simulink model "backwardfault"  (Simulink 8.5)
settings: Solver=ode23tb  SolverMode=SingleTasking  StartTime=0.0  StopTime=0.15  RelTol=1e-3  AbsTol=20e-6
libraries: powerlib x28
settings Model: Creator=Dr. Lotfifard  LastModifiedBy=PC  ExtModeTrigMode=oneshot  ExtModeArmWhenConnect=off
settings SolverCC: MaxOrder=2
settings OptimizationCC: BlockReduction=off  BooleanDataType=off
settings DebuggingCC: SaveWithParameterizedLinksMsg=none  SignalResolutionControl=TryResolveAllWithWarning  MultiTaskDSMMsg=warning  MultiTaskCondExecSysMsg=none  FcnCallInpInsideContextMsg=UseLocalSettings
settings HardwareCC: TargetUnknown=on
settings RTWCC: TemplateMakefile=grt_unix.tmf

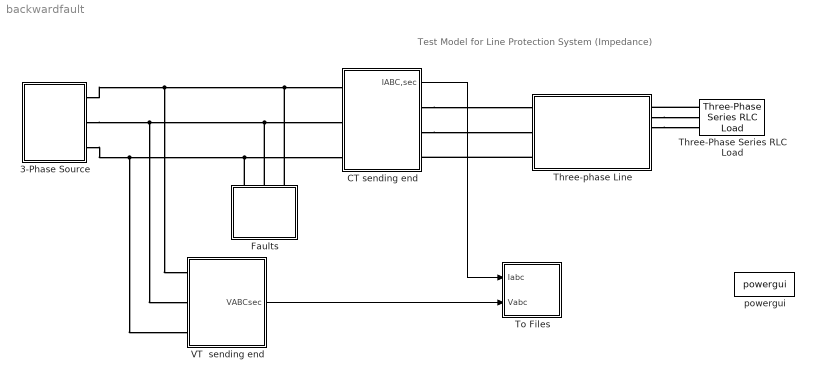
== system backwardfault ==
  note: Test Model for Line Protection System (Impedance)
  3-Phase Source : Subsystem  mask(Three-phase Source){Vrms=1000}
      mask prompts: Vrms "RMS Voltage for each phase"
      mask Display: plot(0,0,100,100,[60,56,50,44,40,36,30,24,20],[50,40,33,40,50,60,66,60,50],[15,20,30,40,50,60,65,60,50,40,30,20,15],[50,35,27,25,26,35,50,65,73,76,73,65,50],[40,40],[90,76],[40,40],[10,25],[60,60],[75,87],[53,67],[79,79])
  CT sending end : Subsystem  mask{TC=1.2}
      mask prompts: TC "Maximum Normal Current"
  Faults : Subsystem  mask{tof='A-G', ft=0.05, RF=1e-6}
      mask prompts: tof "Type of fault"; ft "Fault time (in sec.)"; RF "Fault Resistance RF (in ohms)"
      mask init:
      | switch tof,
      |    case 1,
      |       %No faults or Normal
      |       S1=0;S2=0;S3=0;S4=0;
      |    case 2,
      |       %Fault A-G
      |       S1=1;S2=0;S3=0;S4=1;
      |    case 3,
      |       %Fault B-G
      |       S1=0;S2=1;S3=0;S4=1;
      |    case 4,
      |       %Fault B-G
      |       S1=0;S2=0;S3=1;S4=1;
      |    case 5,
      |       %Fault B-C
      |       S1=0;S2=1;S3=1;S4=0;
      |    case 6,
      |       %Fault A-C
      |       S1=1;S2=0;S3=1;S4=0;
      |    case 7,
      |       %Fault A-B
      |       S1=1;S2=1;S3=0;S4=0;
      |    case 8,
      |       %Fault A-B-C
      |       S1=1;S2=1;S3=1;S4=0;
      |    case 9,
      |       %Fault B-C-G
      |       S1=0;S2=1;S3=1;S4=1;
      |    case 10,
      |       %Fault A-C-G
      |       S1=1;S2=0;S3=1;S4=1;
      |    case 11,
      |       %Fault A-B-G
      |       S1=1;S2=1;S3=0;S4=1;
      |    case 12,
      |       %Fault A-B-C-G
      |       S1=1;S2=1;S3=1;S4=1;
      |    end;
      mask TypeOptions tof: 'Normal' | 'A-G' | 'B-G' | 'C-G' | 'B-C' | 'A-C' | 'A-B' | 'A-B-C' | 'B-C-G' | 'A-C-G' | 'A-B-G' | 'A-B-C-G'
      mask Display: plot(0,0,100,100,[44,47,56,38,50],[23,8,64,44,97],[56,47],[25,8])
  Three-Phase Series RLC Load : powerlib/Elements/Three-Phase Series RLC Load  LConnTagsString=A|B|C  Configuration=Y (grounded)  NominalVoltage=1000  NominalFrequency=60  ActivePower=10e3  InductivePower=100  CapacitivePower=100  Measurements=None  LoadType=constant Z
  Three-phase Line : Subsystem  mask(Three-pase Line){KM=50}
      mask prompts: KM "Fault location (1% to 99%) (the lenght of the line is 100 km):"
      mask Display: plot(0,0,100,100,[20,20,80,80,90,80,80,20,20,10],[50,40,40,50,50,50,61,61,50,50],[56,39],[55,55],[44,44],[44,55],[53,50,50],[44,48,55])
  To Files : Subsystem
  VT  sending end : Subsystem  mask{TP=1000}
      mask prompts: TP "Nominal Voltage,rms"
  powergui : powerlib/powergui  SimulationMode=Continuous  SolverType=Tustin/Backward Euler (TBE)  SampleTime=0  frequency=60  SPID=off  DisableSnubberDevices=off  DisableRonSwitches=off  DisableVfSwitches=off  SwTol=0  DisplayEquations=off  Interpol=off  methode=off  Ts=0  FunctionMessages=off  echomessages=off  HookPort=off  EnableUseOfTLC=off  x0status=blocks  frequencyindice=60  Pbase=100e6  ErrMax=1e-4  Iterations=50  UnitsV=kV  UnitsW=MW  buscounter=0  RestoreLinks=warning  ResistiveCurrentMeasurement=off  Frange=[0:2:500]  Ylog=off  Xlog=on  ShowGrid=off  save=off  variable=ZData  structure=0  ZoomFFT=on  StartTime=0.0  cycles=1  DisplayStyle=1  fundamental=60  FreqAxis=off  MaxFrequency=1000  frequencyindicesteady=1  RmsSteady=1  display=off
  wires:
  CT sending end/1(IABC,sec) -> To Files/1(Iabc)
  VT  sending end/1(VABCsec) -> To Files/2(Vabc)
  connections:
  3-Phase Source/RConn1 -- Faults/LConn3 -- CT sending end/LConn1 -- VT  sending end/LConn1
  3-Phase Source/RConn2 -- Faults/LConn2 -- CT sending end/LConn2 -- VT  sending end/LConn2
  3-Phase Source/RConn3 -- Faults/LConn1 -- CT sending end/LConn3 -- VT  sending end/LConn3
  Three-phase Line/LConn3 -- CT sending end/RConn3
  CT sending end/RConn2 -- Three-phase Line/LConn2
  CT sending end/RConn1 -- Three-phase Line/LConn1
  Three-Phase Series RLC Load/LConn1 -- Three-phase Line/RConn1
  Three-phase Line/RConn2 -- Three-Phase Series RLC Load/LConn2
  Three-phase Line/RConn3 -- Three-Phase Series RLC Load/LConn3

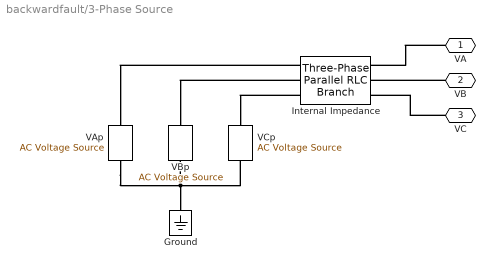
== system backwardfault/3-Phase Source ==
  Ground : powerlib/Elements/Ground  LConnTagsString=a
  Internal Impedance : powerlib/Elements/Three-Phase Parallel RLC Branch  LConnTagsString=A|B|C  RConnTagsString=A|B|C  BranchType=R  Resistance=1  Inductance=1e-3  Capacitance=1e-6  Measurements=None
  VAp : powerlib/Electrical Sources/AC Voltage Source  Amplitude=100  Phase=0  Frequency=60  SampleTime=0  Measurements=None
  VBp : powerlib/Electrical Sources/AC Voltage Source  Amplitude=100  Phase=0  Frequency=60  SampleTime=0  Measurements=None
  VCp : powerlib/Electrical Sources/AC Voltage Source  Amplitude=100  Phase=0  Frequency=60  SampleTime=0  Measurements=None
  VA : PMIOPort  Port=1  Side=Right
  VB : PMIOPort  Port=2  Side=Right
  VC : PMIOPort  Port=3  Side=Right
  connections:
  VAp/LConn1 -- VBp/LConn1 -- Ground/LConn1 -- VCp/LConn1
  Internal Impedance/LConn3 -- VCp/RConn1
  Internal Impedance/LConn2 -- VBp/RConn1
  Internal Impedance/LConn1 -- VAp/RConn1
  VA/RConn1 -- Internal Impedance/RConn1
  VB/RConn1 -- Internal Impedance/RConn2
  VC/RConn1 -- Internal Impedance/RConn3

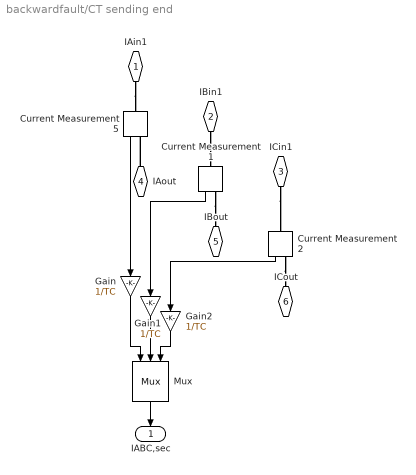
== system backwardfault/CT sending end ==
  Current Measurement1 : powerlib/Measurements/Current Measurement  PhasorSimulation=off  OutputType=Complex  PSBequivalent=0
  Current Measurement2 : powerlib/Measurements/Current Measurement  PhasorSimulation=off  OutputType=Complex  PSBequivalent=0
  Current Measurement5 : powerlib/Measurements/Current Measurement  PhasorSimulation=off  OutputType=Complex  PSBequivalent=0
  Gain : Gain  Gain=1/TC  SaturateOnIntegerOverflow=on  OutDataTypeStr=Inherit: Same as input  ParamDataTypeStr=Inherit: Same as input
  Gain1 : Gain  Gain=1/TC  SaturateOnIntegerOverflow=on  OutDataTypeStr=Inherit: Same as input  ParamDataTypeStr=Inherit: Same as input
  Gain2 : Gain  Gain=1/TC  SaturateOnIntegerOverflow=on  OutDataTypeStr=Inherit: Same as input  ParamDataTypeStr=Inherit: Same as input
  Mux : Mux  Inputs=3
  IAin1 : PMIOPort  Port=1  Side=Left
  IBin1 : PMIOPort  Port=2  Side=Left
  ICin1 : PMIOPort  Port=3  Side=Left
  IAout : PMIOPort  Port=4  Side=Right
  IBout : PMIOPort  Port=5  Side=Right
  ICout : PMIOPort  Port=6  Side=Right
  IABC,sec : Outport  InitialOutput=0
  wires:
  Mux/1 -> IABC,sec/1
  Current Measurement2/1 -> Gain2/1
  Gain/1 -> Mux/1
  Gain1/1 -> Mux/2
  Gain2/1 -> Mux/3
  Current Measurement1/1 -> Gain1/1
  Current Measurement5/1 -> Gain/1
  connections:
  IAin1/RConn1 -- Current Measurement5/LConn1
  ICin1/RConn1 -- Current Measurement2/LConn1
  IBin1/RConn1 -- Current Measurement1/LConn1
  IAout/RConn1 -- Current Measurement5/RConn1
  Current Measurement1/RConn1 -- IBout/RConn1
  Current Measurement2/RConn1 -- ICout/RConn1

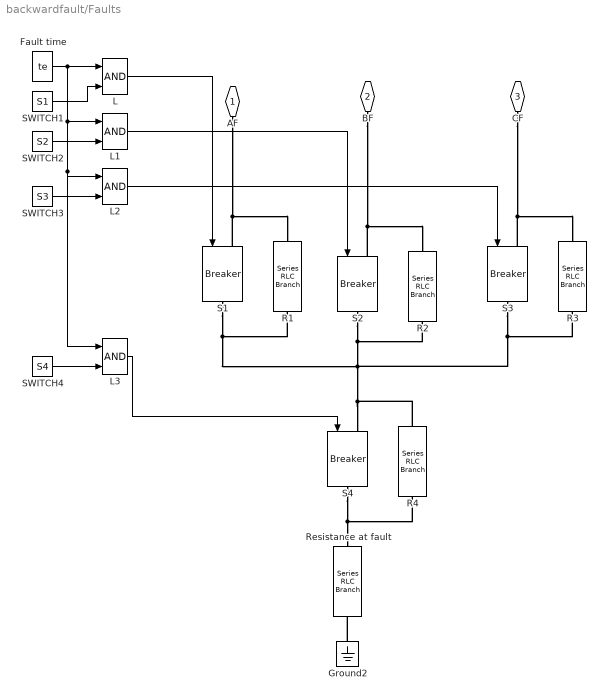
== system backwardfault/Faults ==
  Fault time : FromWorkspace  VariableName=te  SampleTime=0  mask(Fault timing){t=[0 ft 10], e=[0 1 0 ]}
      mask prompts: t "transition steps:"; e "states (0/1):"
      mask help: steps
      mask init:
      | te=[t,t(2:length(t))-1e-8,t(length(t))+1e-8;e,e]';[y,i]=sort(te(:,1));te=[te(i,1),te(i,2)];
      mask Display: plot(te(:,1),te(:,2))
  Ground2 : powerlib/Elements/Ground  LConnTagsString=a
  L{,1..3} (4 alike) : Logic
  R{1..4} (4 alike) : powerlib/Elements/Series RLC Branch  LConnTagsString=__new0  RConnTagsString=__new0  BranchType=R  Resistance=100e6  Inductance=1e-3  SetiL0=off  InitialCurrent=0  Capacitance=1e-6  Setx0=off  InitialVoltage=0  Measurements=None
  Resistance at fault : powerlib/Elements/Series RLC Branch  LConnTagsString=__new0  RConnTagsString=__new0  BranchType=R  Resistance=RF  Inductance=1e-3  SetiL0=off  InitialCurrent=0  Capacitance=1e-6  Setx0=off  InitialVoltage=0  Measurements=None
  S{1..4} (4 alike) : powerlib/Elements/Breaker  InitialState=0  SwitchingTimes="[ 1/60  5/60 ]"  External=on  BreakerResistance=0.01  SnubberResistance=1e6  SnubberCapacitance=inf  Measurements=None  MoreParameters=off  NoBreakLoop=off
  SWITCH1 : Constant  Value=S1
  SWITCH2 : Constant  Value=S2
  SWITCH3 : Constant  Value=S3
  SWITCH4 : Constant  Value=S4
  AF : PMIOPort  Port=1  Side=Left
  BF : PMIOPort  Port=2  Side=Left
  CF : PMIOPort  Port=3  Side=Left
  wires:
  Fault time/1 -> L/1, L1/1, L2/1, L3/1
  SWITCH1/1 -> L/2
  SWITCH2/1 -> L1/2
  SWITCH3/1 -> L2/2
  L/1 -> S1/1
  SWITCH4/1 -> L3/2
  L1/1 -> S2/1
  L2/1 -> S3/1
  L3/1 -> S4/1
  connections:
  S1/LConn1 -- R1/RConn1 -- AF/RConn1
  BF/RConn1 -- S2/LConn1 -- R2/RConn1
  CF/RConn1 -- S3/LConn1 -- R3/RConn1
  S1/RConn1 -- S2/RConn1 -- R2/LConn1 -- R4/RConn1 -- S4/LConn1 -- S3/RConn1 -- R3/LConn1 -- R1/LConn1
  S4/RConn1 -- R4/LConn1 -- Resistance at fault/LConn1
  Ground2/LConn1 -- Resistance at fault/RConn1

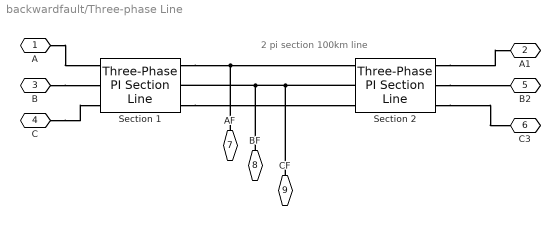
== system backwardfault/Three-phase Line ==
  note: 2 pi section 100km line
  Section 1 : powerlib/Elements/Three-Phase PI Section Line  LConnTagsString=a|b|c  RConnTagsString=A|B|C  Frequency=60  Resistances=[0.01273 0.3864]  Inductances="[0.9337e-3  4.1264e-3]"  Capacitances=[12.74e-9 7.751e-9]  Length=100
  Section 2 : powerlib/Elements/Three-Phase PI Section Line  LConnTagsString=a|b|c  RConnTagsString=A|B|C  Frequency=60  Resistances=[0.01273 0.3864]  Inductances="[0.9337e-3  4.1264e-3]"  Capacitances=[12.74e-9 7.751e-9]  Length=100
  A : PMIOPort  Port=1  Side=Left
  A1 : PMIOPort  Port=2  Side=Right
  B : PMIOPort  Port=3  Side=Left
  C : PMIOPort  Port=4  Side=Left
  B2 : PMIOPort  Port=5  Side=Right
  C3 : PMIOPort  Port=6  Side=Right
  AF : PMIOPort  Port=7  Side=Right
  BF : PMIOPort  Port=8  Side=Right
  CF : PMIOPort  Port=9  Side=Right
  connections:
  Section 2/RConn1 -- A1/RConn1
  Section 2/RConn2 -- B2/RConn1
  Section 2/RConn3 -- C3/RConn1
  Section 1/RConn1 -- Section 2/LConn1 -- AF/RConn1
  Section 2/LConn2 -- Section 1/RConn2 -- BF/RConn1 -- CF/RConn1
  Section 1/RConn3 -- Section 2/LConn3
  A/RConn1 -- Section 1/LConn1
  B/RConn1 -- Section 1/LConn2
  C/RConn1 -- Section 1/LConn3

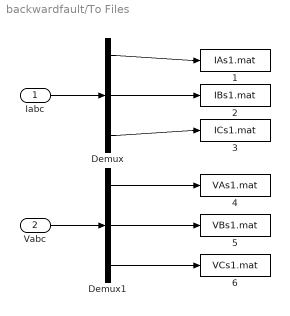
== system backwardfault/To Files ==
  Iabc : Inport
  Vabc : Inport  Port=2
  1 : ToFile  Filename=IAs1.mat
  2 : ToFile  Filename=IBs1.mat
  3 : ToFile  Filename=ICs1.mat
  4 : ToFile  Filename=VAs1.mat
  5 : ToFile  Filename=VBs1.mat
  6 : ToFile  Filename=VCs1.mat
  Demux : Demux  Outputs=3
  Demux1 : Demux  Outputs=3
  wires:
  Demux/2 -> 2/1
  Demux1/1 -> 4/1
  Demux1/2 -> 5/1
  Demux/1 -> 1/1
  Demux/3 -> 3/1
  Demux1/3 -> 6/1
  Iabc/1 -> Demux/1
  Vabc/1 -> Demux1/1

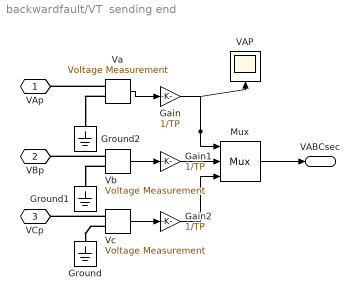
== system backwardfault/VT  sending end ==
  Gain : Gain  Gain=1/TP  SaturateOnIntegerOverflow=on  OutDataTypeStr=Inherit: Same as input  ParamDataTypeStr=Inherit: Same as input
  Gain1 : Gain  Gain=1/TP  SaturateOnIntegerOverflow=on  OutDataTypeStr=Inherit: Same as input  ParamDataTypeStr=Inherit: Same as input
  Gain2 : Gain  Gain=1/TP  SaturateOnIntegerOverflow=on  OutDataTypeStr=Inherit: Same as input  ParamDataTypeStr=Inherit: Same as input
  Ground : powerlib/Elements/Ground  LConnTagsString=a
  Ground1 : powerlib/Elements/Ground  LConnTagsString=a
  Ground2 : powerlib/Elements/Ground  LConnTagsString=a
  Mux : Mux  Inputs=3
  VAP : Scope
      settings: TickLabels=on  YMin=-1.5  YMax=1.75
  Va : powerlib/Measurements/Voltage Measurement  PhasorSimulation=off  OutputType=Complex  PSBequivalent=0
  Vb : powerlib/Measurements/Voltage Measurement  PhasorSimulation=off  OutputType=Complex  PSBequivalent=0
  Vc : powerlib/Measurements/Voltage Measurement  PhasorSimulation=off  OutputType=Complex  PSBequivalent=0
  VAp : PMIOPort  Port=1  Side=Left
  VBp : PMIOPort  Port=2  Side=Left
  VCp : PMIOPort  Port=3  Side=Left
  VABCsec : Outport
  wires:
  Gain1/1 -> Mux/2
  Vb/1 -> Gain1/1
  Mux/1 -> VABCsec/1
  Gain2/1 -> Mux/3
  Vc/1 -> Gain2/1
  Va/1 -> Gain/1
  Gain/1 -> Mux/1, VAP/1
  connections:
  Vc/LConn2 -- Ground/LConn1
  Vb/LConn2 -- Ground1/LConn1
  Va/LConn2 -- Ground2/LConn1
  Va/LConn1 -- VAp/RConn1
  Vb/LConn1 -- VBp/RConn1
  Vc/LConn1 -- VCp/RConn1
